simulink model "RL_Renewable_energy_smoothing_2023b"  (R2023b)
settings: Solver=VariableStepAuto  StartTime=0.0  StopTime=50  FixedStep=0.01  RelTol=1e-3
InitFcn:
  | SP_CH=1;
  | TECH_EXP=0;
  | TECH_Pro=0.5;
undefined symbols (not defined in the file or in its folder): Ts
libraries: simulink x8, spsMeanLib x1, slpidlib x1, rllib x1
settings Model: Creator=User  LastModifiedBy=User
settings RTWCC: GPUComputeCapability=5.0

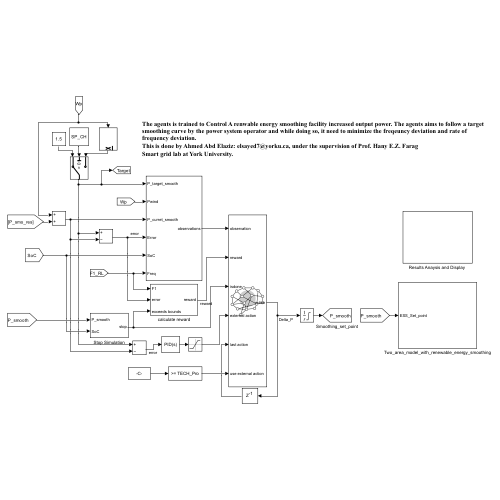
[thumbnail: Simulink's stored preview of the top-level diagram]
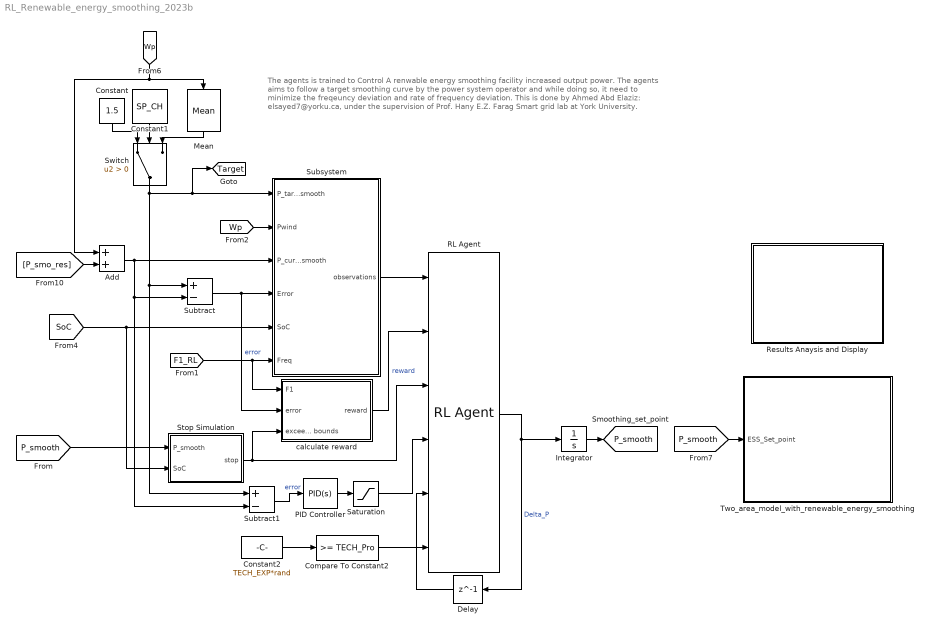
== system RL_Renewable_energy_smoothing_2023b ==
  note: The agents is trained to Control A renwable energy smoothing facility increased output power. The agents aims to follow a target smoothing curve by the power system operator and while doing so, it need to minimize the freqeuncy deviation and rate of frequency deviation.
      | This is done by Ahmed Abd Elaziz: elsayed7@yorku.ca, under the supervision of Prof. Hany E.Z. Farag
      | Smart grid lab at York University.
  Add : Sum
  Compare To Constant2 : simulink/Logic and Bit Operations/Compare To Constant  relop=>=  const=TECH_Pro  OutDataTypeStr=boolean
  Constant : Constant  Value=1.5
  Constant1 : Constant  Value=SP_CH
  Constant2 : Constant  Value=TECH_EXP*rand
  Delay : Delay  DelayLength=1  InitialCondition=0  SampleTime=Ts
  Integrator : Integrator  LimitOutput=on  UpperSaturationLimit=0.1  LowerSaturationLimit=-0.1
  Mean : spsMeanLib/Mean  Freq=1/6  Vinit=1.6  Ts=Ts
  PID Controller : slpidlib/PID Controller  Controller=PID  Form=Parallel  TimeDomain=Continuous-time  UseExternalTs=off  SampleTime=-1  IntegratorMethod=Forward Euler  FilterMethod=Forward Euler  ControllerParametersSource=internal  P=0.9  I=0.4  UseKiTs=off  D=0  N=100  UseFilter=on  TunerSelectOption=Transfer Function Based (PID Tuner App)  InitialConditionSource=internal  InitialConditionForIntegrator=0  InitialConditionForFilter=0  DifferentiatorICPrevScaledInput=0  ExternalReset=none  TrackingMode=off  Kt=1  LimitOutput=off  SatLimitsSource=internal  UpperSaturationLimit=inf  LowerSaturationLimit=-inf  LinearizeAsGain=on  AntiWindupMode=none  Kb=1  LimitIntegrator=off  UpperIntegratorSaturationLimit=inf  LowerIntegratorSaturationLimit=-inf  POutMin=[]  POutMax=[]  IOutMin=[]  IOutMax=[]  DOutMin=[]  DOutMax=[]  NOutMin=[]  NOutMax=[]  SumOutMin=[]  SumOutMax=[]  SaturationOutMin=[]  SaturationOutMax=[]  PParamMin=[]  PParamMax=[]  IParamMin=[]  IParamMax=[]  DParamMin=[]  DParamMax=[]  NParamMin=[]  NParamMax=[]  KbParamMin=[]  KbParamMax=[]  KtParamMin=[]  KtParamMax=[]  KbOutMin=[]  KbOutMax=[]  KtOutMin=[]  KtOutMax=[]  IntegratorOutMin=[]  IntegratorOutMax=[]  FilterOutMin=[]  FilterOutMax=[]  SumI1OutMin=[]  SumI1OutMax=[]  SumI2OutMin=[]  SumI2OutMax=[]  SumI3OutMin=[]  SumI3OutMax=[]  SumI4OutMin=[]  SumI4OutMax=[]  SumDOutMin=[]  SumDOutMax=[]  DifferentiatorOutMin=[]  DifferentiatorOutMax=[]  FilterDiffOutCoefMin=[]  FilterDiffOutCoefMax=[]  ReciprocalOutMin=[]  ReciprocalOutMax=[]  SumDenOutMin=[]  SumDenOutMax=[]  SumNumOutMin=[]  SumNumOutMax=[]  DivideOutMin=[]  DivideOutMax=[]  UdiffTsProdOutMin=[]  UdiffTsProdOutMax=[]  NTsProdOutMin=[]  NTsProdOutMax=[]  UintegralTsProdOutMin=[]  UintegralTsProdOutMax=[]  UngainTsProdOutMin=[]  UngainTsProdOutMax=[]  ClampingZeroOutDataTypeStr=Inherit: Inherit via back propagation  ClampingZeroOutMin=[]  ClampingZeroOutMax=[]  FilterDenConstantOutDataTypeStr=Inherit: Inherit via back propagation  FilterDenConstantOutMin=[]  FilterDenConstantOutMax=[]  PCopyOutDataTypeStr=Inherit: Inherit via back propagation  PCopyOutMin=[]  PCopyOutMax=[]  NCopyOutDataTypeStr=Inherit: Inherit via back propagation  NCopyOutMin=[]  NCopyOutMax=[]  IntegratorContinuousStateAttributes=''  IntegratorStateMustResolveToSignalObject=off  IntegratorRTWStateStorageClass=Auto  FilterContinuousStateAttributes=''  FilterStateMustResolveToSignalObject=off  FilterRTWStateStorageClass=Auto  ParallelPVariant=InternalParameters  IdealPVariant=Disabled  IVariant=InternalParameters  DVariant=InternalParameters  IntegratorVariant=Continuous  SatVariant=Disabled  AWVariant=Passthrough  PCopyVariant=Disabled  TRVariant=Disabled  FdbkBlocksVariant=Forward  IdealPFdbkVariant=Disabled  SatFdbkVariant=Disabled  DerivativeFilterVariant=ContFilter  NVariant=InternalParameters  NCopyVariant=Disabled  FilterICVariant=InternalICsFilter  IntegratorICVariant=InternalICs  ExternalResetVariant=Disabled  TRSumVariant=Passthrough  SumFdbkVariant=Disabled  SumVariant=Sum_PID  TsampFilterVariant=InternalTs  TsampNgainVariant=Passthrough  TsampIntegralVariant=Disabled_SignalSpec  ExternalSaturationOutDataTypeStr=Inherit: Same as second input
  RL Agent : rllib/RL Agent  Agent=agent  ExternalActionAsInput=on  ProvideLastAction=on  ProvideCumRwd=off  TreatAsDirectFeedthrough=on  UseStrictObservationDataTypes=off
  "Results Anaysis and Display " : Subsystem
  Saturation : Saturate  UpperLimit=0.1  LowerLimit=-0.1
  Stop Simulation : Subsystem
  Subsystem : Subsystem
  Subtract : Sum  Inputs=+-
  Subtract1 : Sum  Inputs=+-
  Switch : Switch  Criteria=u2 > Threshold  SaturateOnIntegerOverflow=off  InputSameDT=off
  Two_area_model_with_renewable_energy_smoothing : Subsystem
  calculate reward : Subsystem
  tag scope: P_smooth=global, Target=global
  wires:
  [P_smooth] -> Stop Simulation/1(P_smooth)
  [P_smo_res] -> Add/2
  Stop Simulation/1(stop) -> calculate reward/3(exceeds bounds), RL Agent/3
  [F1_RL] -> calculate reward/1(F1), Subsystem/6(Freq)
  Subtract/1 -> calculate reward/2(error), Subsystem/4(Error)  "error"
  RL Agent/1 -> Integrator/1, Delay/1  "Delta_P"
  Subsystem/1(observations) -> RL Agent/1
  calculate reward/1(reward) -> RL Agent/2  "reward"
  Compare To Constant2/1 -> RL Agent/6
  Add/1 -> Subtract/2, Subtract1/2, Subsystem/3(P_curret_smooth)
  Subtract1/1 -> PID Controller/1  "error"
  Integrator/1 -> [P_smooth]
  PID Controller/1 -> Saturation/1
  Constant2/1 -> Compare To Constant2/1
  [Wp] -> Mean/1, Add/1
  Mean/1 -> Switch/3
  Constant1/1 -> Switch/2
  Switch/1 -> Subtract/1, Subtract1/1, [Target], Subsystem/1(P_target_smooth)
  [Wp] -> Subsystem/2(Pwind)
  Constant/1 -> Switch/1
  [P_smooth] -> Two_area_model_with_renewable_energy_smoothing/1(ESS_Set_point)
  [SoC] -> Subsystem/5(SoC), Stop Simulation/2(SoC)
  Saturation/1 -> RL Agent/4
  Delay/1 -> RL Agent/5

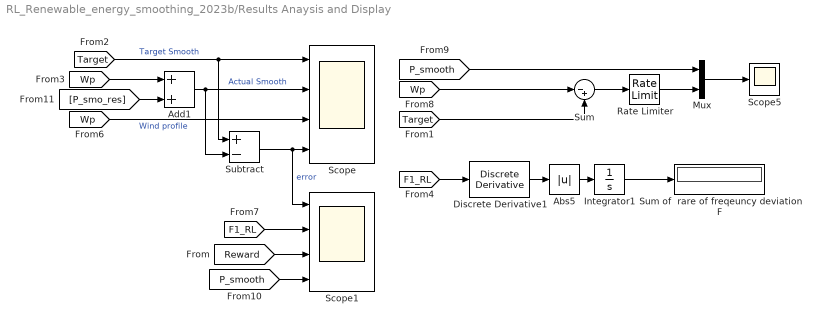
== system RL_Renewable_energy_smoothing_2023b/Results Anaysis and Display  ==
  Abs5 : Abs  SaturateOnIntegerOverflow=off
  Add1 : Sum
  Discrete Derivative1 : simulink/Discrete/Discrete Derivative  gainval=1.0  ICPrevScaledInput=0.0  OutMin=[]  OutMax=[]  OutDataType=fixdt(1, 16)  OutScaling=2^-10  DoSatur=off
  Integrator1 : Integrator
  Mux : Mux  Inputs=2
  Rate Limiter : RateLimiter  RisingSlewLimit=0.1  FallingSlewLimit=-0.1  SampleTimeMode=inherited
  Scope : Scope  NumInputPorts=4
  Scope1 : Scope  NumInputPorts=4
  Scope5 : Scope
  Subtract : Sum  Inputs=+-
  Sum : Sum  Inputs=|-+
  Sum of  rare of freqeuncy deviation F : Display
  wires:
  Rate Limiter/1 -> Mux/2
  Mux/1 -> Scope5/1
  Sum/1 -> Rate Limiter/1
  [Target] -> Sum/2
  [Wp] -> Sum/1
  [P_smooth] -> Mux/1
  Abs5/1 -> Integrator1/1
  Integrator1/1 -> Sum of  rare of freqeuncy deviation F/1
  [F1_RL] -> Discrete Derivative1/1
  Discrete Derivative1/1 -> Abs5/1
  [P_smo_res] -> Add1/2
  [Target] -> Scope/1, Subtract/1  "Target Smooth"
  [Wp] -> Add1/1
  Add1/1 -> Subtract/2, Scope/2  "Actual Smooth"
  [Wp] -> Scope/3  "Wind profile"
  Subtract/1 -> Scope1/1, Scope/4  "error"
  [F1_RL] -> Scope1/2
  [Reward] -> Scope1/3
  [P_smooth] -> Scope1/4

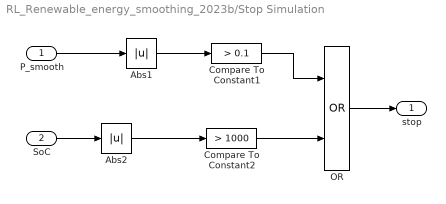
== system RL_Renewable_energy_smoothing_2023b/Stop Simulation ==
  P_smooth : Inport
  SoC : Inport  Port=2
  Abs1 : Abs  SaturateOnIntegerOverflow=off
  Abs2 : Abs  SaturateOnIntegerOverflow=off
  Compare To Constant1 : simulink/Logic and Bit Operations/Compare To Constant  relop=>  const=0.1  OutDataTypeStr=boolean
  Compare To Constant2 : simulink/Logic and Bit Operations/Compare To Constant  relop=>  const=1000  OutDataTypeStr=boolean
  OR : Logic  Operator=OR  IconShape=distinctive  AllPortsSameDT=off  OutDataTypeStr=boolean
  stop : Outport  VectorParamsAs1DForOutWhenUnconnected=off
  wires:
  P_smooth/1 -> Abs1/1
  OR/1 -> stop/1
  Compare To Constant1/1 -> OR/1
  Abs1/1 -> Compare To Constant1/1
  SoC/1 -> Abs2/1
  Abs2/1 -> Compare To Constant2/1
  Compare To Constant2/1 -> OR/2

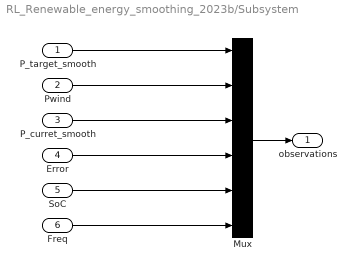
== system RL_Renewable_energy_smoothing_2023b/Subsystem ==
  P_target_smooth : Inport
  Pwind : Inport  Port=2
  P_curret_smooth : Inport  Port=3
  Error : Inport  Port=4
  SoC : Inport  Port=5
  Freq : Inport  Port=6
  Mux : Mux  Inputs=6
  observations : Outport  VectorParamsAs1DForOutWhenUnconnected=off
  wires:
  Mux/1 -> observations/1
  P_target_smooth/1 -> Mux/1
  Error/1 -> Mux/4
  P_curret_smooth/1 -> Mux/3
  Pwind/1 -> Mux/2
  SoC/1 -> Mux/5
  Freq/1 -> Mux/6

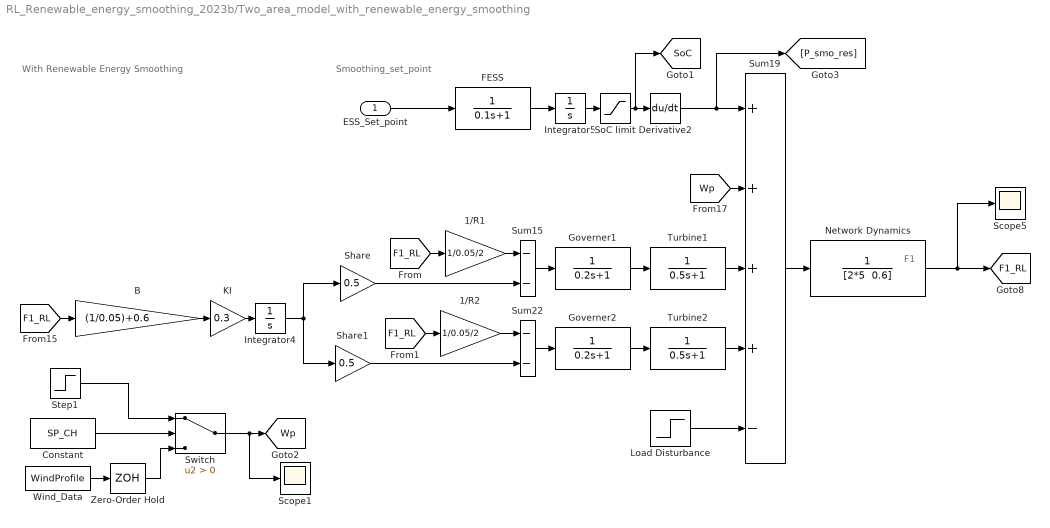
== system RL_Renewable_energy_smoothing_2023b/Two_area_model_with_renewable_energy_smoothing ==
  note: Smoothing_set_point
  note: With Renewable Energy Smoothing
  note: F1
  ESS_Set_point : Inport
  1/R1 : Gain  Gain=1/0.05/2
  1/R2 : Gain  Gain=1/0.05/2
  B : Gain  Gain=(1/0.05)+0.6
  Constant : Constant  Value=SP_CH
  Derivative2 : Derivative
  FESS : TransferFcn  Numerator=[0 1]  Denominator="[0.1  1]"
  Governer1 : TransferFcn  Numerator=[0 1]  Denominator="[0.2  1]"
  Governer2 : TransferFcn  Numerator=[0 1]  Denominator="[0.2  1]"
  Integrator4 : Integrator
  Integrator5 : Integrator  InitialCondition=-9600/10/2
  KI : Gain  Gain=0.3
  Load Disturbance : Step  Time=20+rand*10
  Network Dynamics : TransferFcn  Denominator="[2*5  0.6]"
  Scope1 : Scope
  Scope5 : Scope
  Share : Gain  Gain=0.5
  Share1 : Gain  Gain=0.5
  SoC limit : Saturate  UpperLimit=0  LowerLimit=-9600/10
  Step1 : Step  Time=25  Before=1.5  After=1.55  SampleTime=0
  Sum15 : Sum  Inputs=--  InputSameDT=on  SaturateOnIntegerOverflow=on  OutDataTypeStr=Inherit: Same as first input
  Sum19 : Sum  Inputs=++++-  InputSameDT=on  SaturateOnIntegerOverflow=on  OutDataTypeStr=Inherit: Same as first input
  Sum22 : Sum  Inputs=--  InputSameDT=on  SaturateOnIntegerOverflow=on  OutDataTypeStr=Inherit: Same as first input
  Switch : Switch  Criteria=u2 > Threshold  SaturateOnIntegerOverflow=off  InputSameDT=off
  Turbine1 : TransferFcn  Numerator=[0 1]  Denominator="[0.5  1]"
  Turbine2 : TransferFcn  Numerator=[0 1]  Denominator="[0.5  1]"
  Wind_Data : FromWorkspace  VariableName=WindProfile  SampleTime=0.1
  Zero-Order Hold : ZeroOrderHold  SampleTime=0.01
  tag scope: F1_RL=global, SoC=global, Wp=global
  wires:
  Wind_Data/1 -> Zero-Order Hold/1
  Switch/1 -> Scope1/1, [Wp]
  Zero-Order Hold/1 -> Switch/3
  Constant/1 -> Switch/2
  Step1/1 -> Switch/1
  1/R2/1 -> Sum22/1
  Network Dynamics/1 -> Scope5/1, [F1_RL]
  Governer2/1 -> Turbine2/1
  Integrator5/1 -> SoC limit/1
  KI/1 -> Integrator4/1
  Sum22/1 -> Governer2/1
  Share1/1 -> Sum22/2
  [F1_RL] -> B/1
  [F1_RL] -> 1/R2/1
  Governer1/1 -> Turbine1/1
  1/R1/1 -> Sum15/1
  Turbine1/1 -> Sum19/3
  B/1 -> KI/1
  FESS/1 -> Integrator5/1
  Share/1 -> Sum15/2
  SoC limit/1 -> Derivative2/1, [SoC]
  Sum19/1 -> Network Dynamics/1
  Integrator4/1 -> Share1/1, Share/1
  Load Disturbance/1 -> Sum19/5
  Sum15/1 -> Governer1/1
  Derivative2/1 -> [P_smo_res], Sum19/1
  Turbine2/1 -> Sum19/4
  [Wp] -> Sum19/2
  ESS_Set_point/1 -> FESS/1
  [F1_RL] -> 1/R1/1

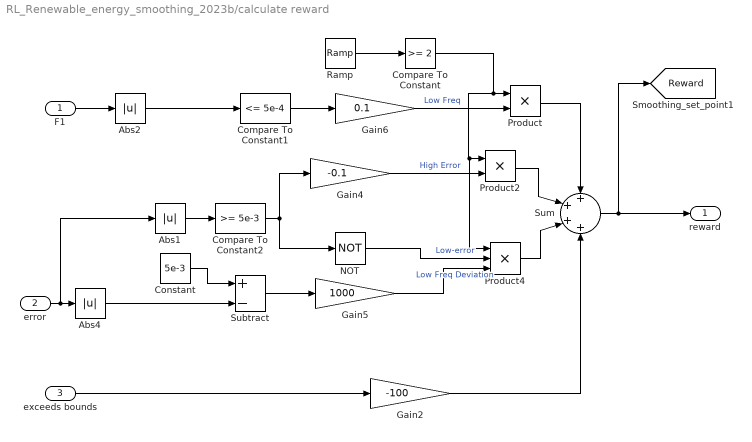
== system RL_Renewable_energy_smoothing_2023b/calculate reward ==
  F1 : Inport
  error : Inport  Port=2
  exceeds bounds : Inport  Port=3
  Abs1 : Abs  SaturateOnIntegerOverflow=off
  Abs2 : Abs  SaturateOnIntegerOverflow=off
  Abs4 : Abs  SaturateOnIntegerOverflow=off
  Compare To Constant : simulink/Logic and Bit Operations/Compare To Constant  relop=>=  const=2  OutDataTypeStr=boolean
  Compare To Constant1 : simulink/Logic and Bit Operations/Compare To Constant  relop=<=  const=5e-4  OutDataTypeStr=boolean
  Compare To Constant2 : simulink/Logic and Bit Operations/Compare To Constant  relop=>=  const=5e-3  OutDataTypeStr=boolean
  Constant : Constant  Value=5e-3
  Gain2 : Gain  Gain=-100
  Gain4 : Gain  Gain=-0.1
  Gain5 : Gain  Gain=1000
  Gain6 : Gain  Gain=0.1
  NOT : Logic  Operator=NOT  IconShape=distinctive  AllPortsSameDT=off  OutDataTypeStr=boolean
  Product : Product
  Product2 : Product
  Product4 : Product  Inputs=3
  Ramp : simulink/Sources/Ramp  slope=1  start=0  InitialOutput=0
  Subtract : Sum  Inputs=+-
  Sum : Sum  Inputs=++++  OutDataTypeStr=double
  reward : Outport  VectorParamsAs1DForOutWhenUnconnected=off
  tag scope: Reward=global
  wires:
  Sum/1 -> [Reward], reward/1
  exceeds bounds/1 -> Gain2/1
  F1/1 -> Abs2/1
  error/1 -> Abs1/1, Abs4/1
  Ramp/1 -> Compare To Constant/1
  Compare To Constant1/1 -> Gain6/1
  Product/1 -> Sum/1
  Compare To Constant/1 -> Product/1, Product4/1, Product2/1
  Gain4/1 -> Product2/2  "High Error"
  Abs1/1 -> Compare To Constant2/1
  Compare To Constant2/1 -> Gain4/1, NOT/1
  NOT/1 -> Product4/2  "Low-error"
  Constant/1 -> Subtract/1
  Gain5/1 -> Product4/3  "Low Freq Deviation"
  Subtract/1 -> Gain5/1
  Abs2/1 -> Compare To Constant1/1
  Gain6/1 -> Product/2  "Low Freq"
  Abs4/1 -> Subtract/2
  Gain2/1 -> Sum/4
  Product2/1 -> Sum/2
  Product4/1 -> Sum/3
